simulink model "practicauno"  (R2024b)
settings: Solver=VariableStepAuto  StartTime=0.0  StopTime=10  RelTol=1e-3
InitFcn:
  | Ip=0.0079;
  | Mc=0.7031;
  | Lp=0.3302;
  | Mp=0.23;
  | Fc=0;
  | Beq=4.3;
  | g=9.81;
  | Bp=0.0024;

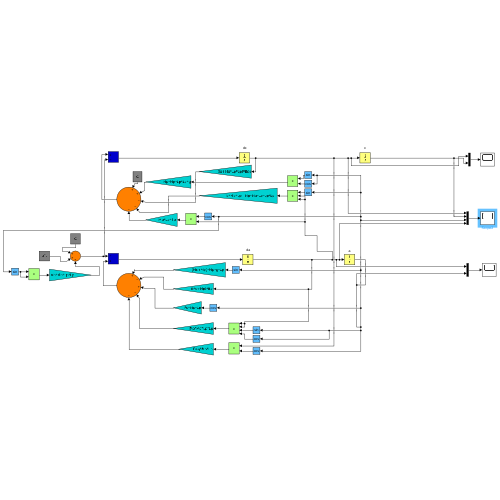
[thumbnail: Simulink's stored preview of the top-level diagram]
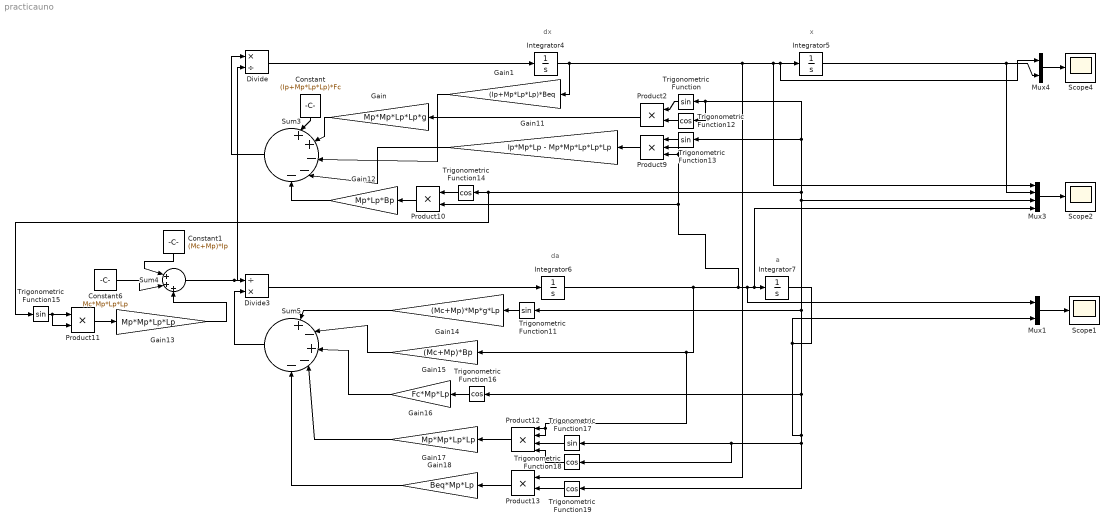
== system practicauno ==
  note: x
  note: dx
  note: da
  note: a
  Constant : Constant  Value=(Ip+Mp*Lp*Lp)*Fc
  Constant1 : Constant  Value=(Mc+Mp)*Ip
  Constant6 : Constant  Value=Mc*Mp*Lp*Lp
  Divide : Product  Inputs=*/
  Divide3 : Product  Inputs=/*
  Gain : Gain  Gain=Mp*Mp*Lp*Lp*g
  Gain1 : Gain  Gain=(Ip+Mp*Lp*Lp)*Beq
  Gain11 : Gain  Gain=Ip*Mp*Lp - Mp*Mp*Lp*Lp*Lp
  Gain12 : Gain  Gain=Mp*Lp*Bp
  Gain13 : Gain  Gain=Mp*Mp*Lp*Lp
  Gain14 : Gain  Gain=(Mc+Mp)*Mp*g*Lp
  Gain15 : Gain  Gain=(Mc+Mp)*Bp
  Gain16 : Gain  Gain=Fc*Mp*Lp
  Gain17 : Gain  Gain=Mp*Mp*Lp*Lp
  Gain18 : Gain  Gain=Beq*Mp*Lp
  Integrator4 : Integrator
  Integrator5 : Integrator
  Integrator6 : Integrator
  Integrator7 : Integrator  InitialCondition=pi/180
  Mux1 : Mux  Inputs=2
  Mux3 : Mux
  Mux4 : Mux  Inputs=2
  Product{2,10..11,13} (4 alike) : Product
  Product12 : Product  Inputs=4
  Product9 : Product  Inputs=3
  Scope1 : Scope
  Scope2 : Scope
  Scope4 : Scope
  Sum3 : Sum  Inputs=|+|+|-|-|-
  Sum4 : Sum  Inputs=|+++
  Sum5 : Sum  Inputs=|+|-|+|-|-
  Trigonometric Function{,11,13,15,17} (5 alike) : Trigonometry
  Trigonometric Function{12,14,16,18..19} (5 alike) : Trigonometry  Operator=cos
  wires:
  Gain13/1 -> Sum4/3
  Trigonometric Function/1 -> Product2/1
  Sum4/1 -> Divide3/1, Divide/2
  Product2/1 -> Gain/1
  Trigonometric Function18/1 -> Product12/4
  Trigonometric Function19/1 -> Product13/2
  Integrator4/1 -> Mux3/1, Mux4/1, Integrator5/1, Product13/1, Gain1/1
  Gain12/1 -> Sum3/5
  Trigonometric Function17/1 -> Product12/3
  Gain11/1 -> Sum3/4
  Trigonometric Function13/1 -> Product9/1
  Gain17/1 -> Sum5/4
  Gain16/1 -> Sum5/3
  Trigonometric Function15/1 -> Product11/2, Product11/1
  Trigonometric Function11/1 -> Gain14/1
  Gain/1 -> Sum3/2
  Gain1/1 -> Sum3/3
  Trigonometric Function12/1 -> Product2/2
  Constant/1 -> Sum3/1
  Product10/1 -> Gain12/1
  Gain15/1 -> Sum5/2
  Gain18/1 -> Sum5/5
  Constant1/1 -> Sum4/1
  Constant6/1 -> Sum4/2
  Integrator5/1 -> Mux3/2, Mux4/2
  Product12/1 -> Gain17/1
  Gain14/1 -> Sum5/1
  Trigonometric Function14/1 -> Product10/1
  Sum3/1 -> Divide/1
  Trigonometric Function16/1 -> Gain16/1
  Mux4/1 -> Scope4/1
  Integrator6/1 -> Product12/2, Product12/1, Gain15/1, Mux1/1, Mux3/4, Integrator7/1, Product9/2, Product9/3, Product10/2
  Mux1/1 -> Scope1/1
  Integrator7/1 -> Trigonometric Function16/1, Trigonometric Function11/1, Trigonometric Function12/1, Trigonometric Function/1, Trigonometric Function13/1, Trigonometric Function15/1, Trigonometric Function14/1, Mux3/3, Trigonometric Function19/1, Trigonometric Function18/1, Trigonometric Function17/1, Mux1/2
  Mux3/1 -> Scope2/1
  Product9/1 -> Gain11/1
  Sum5/1 -> Divide3/2
  Product13/1 -> Gain18/1
  Product11/1 -> Gain13/1
  Divide/1 -> Integrator4/1
  Divide3/1 -> Integrator6/1
